simulink model "VV_Look"  (R2018b)
settings: Solver=VariableStepAuto  StartTime=0.0  StopTime=10.0  RelTol=1e-3
settings Model: Creator=kekos  LastModifiedBy=kekos

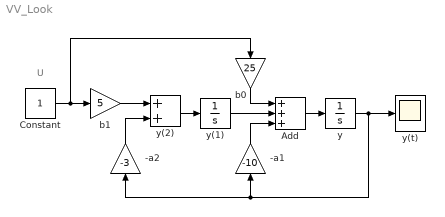
== system VV_Look ==
  note: U
  -a1 : Gain  Gain=-10
  -a2 : Gain  Gain=-3
  Add : Sum  Inputs=3
  Constant : Constant
  b0 : Gain  Gain=25
  b1 : Gain  Gain=5
  y : Integrator  InitialCondition=0.3
  y(1) : Integrator  InitialCondition=3.4
  y(2) : Sum  Inputs=2
  y(t) : Scope
  wires:
  y/1 -> -a2/1, -a1/1, y(t)/1
  -a1/1 -> Add/3
  Constant/1 -> b0/1, b1/1
  b0/1 -> Add/1
  Add/1 -> y/1
  y(2)/1 -> y(1)/1
  -a2/1 -> y(2)/2
  b1/1 -> y(2)/1
  y(1)/1 -> Add/2
